simulink model "subsampling2"  (R2021a)
settings: Solver=VariableStepAuto  StartTime=0.0  StopTime=1  MaxStep=1/1e6  RelTol=1e-3
values from neighbouring files (symbols this model uses):
  fnoise = 1e6    (= 1000000)    [subsampling_1.m]    (also in subsampling_2.m; subsampling_3.m = 3000000; unterabtastung_1.m; unterabtastung_2.m)
  fs = 18e3    (= 18000)    [subsampling_1.m]    (also in subsampling_2.m; subsampling_3.m = 450000; unterabtastung_1.m; unterabtastung_2.m)
  fsin = 39e3    (= 39000)    [subsampling_1.m]    (also in subsampling_2.m; subsampling_3.m = 980000; unterabtastung_1.m; unterabtastung_2.m)
undefined symbols (not defined in the file or in its folder): a, b
libraries: simulink x1, dspstat3 x1, dspsigops x1
settings Model: Creator=josef  LastModifiedBy=josef
settings SolverCC: AlgebraicLoopSolver=TrustRegion
settings DataIOCC: ReturnWorkspaceOutputs=off
settings DebuggingCC: SFMachineParentedDataDiag=warning

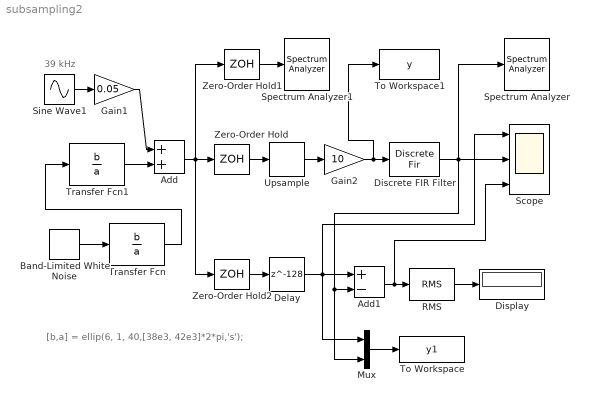
== system subsampling2 ==
  note: [b,a] = ellip(6, 1, 40,[38e3, 42e3]*2*pi,'s');
  note: 39 kHz
  Add : Sum
  Add1 : Sum  Inputs=+-
  Band-Limited White Noise : simulink/Sources/Band-Limited White Noise  Cov=1/fnoise  Ts=1/fnoise  seed=[23341]
  Delay : Delay  DelayLength=128
  Discrete FIR Filter : DiscreteFir  Coefficients=fir1(256,[36, 44]*2e3/(fs*10))
  Display : Display
  Gain1 : Gain  Gain=0.05
  Gain2 : Gain  Gain=10
  Mux : Mux  Inputs=2
  RMS : dspstat3/RMS  run=on  directionMode=Each column  dimension=1  InputProcessing=Columns as channels (frame based)  reset_popup=None
  Scope : Scope  NumInputPorts=3
  Sine Wave1 : Sin  Frequency=2*pi*fsin  SampleTime=0
  Spectrum Analyzer : SpectrumAnalyzer
  Spectrum Analyzer1 : SpectrumAnalyzer
  To Workspace : ToWorkspace  VariableName=y1  SaveFormat=Timeseries  SampleTime=-1
  To Workspace1 : ToWorkspace  VariableName=y  SaveFormat=Timeseries  SampleTime=-1
  Transfer Fcn : TransferFcn  Numerator=b  Denominator=a
  Transfer Fcn1 : TransferFcn  Numerator=b  Denominator=a
  Upsample : dspsigops/Upsample  N=10  phase=0  RateOptions=Allow multirate processing  ic=0  mode=Unused parameter value
  Zero-Order Hold : ZeroOrderHold  SampleTime=1/fs
  Zero-Order Hold1 : ZeroOrderHold  SampleTime=1/(10*fs)
  Zero-Order Hold2 : ZeroOrderHold  SampleTime=1/(10*fs)
  wires:
  Sine Wave1/1 -> Gain1/1
  Add/1 -> Zero-Order Hold2/1, Zero-Order Hold1/1, Zero-Order Hold/1
  Gain1/1 -> Add/1
  Zero-Order Hold/1 -> Upsample/1
  Zero-Order Hold1/1 -> Spectrum Analyzer1/1
  Band-Limited White Noise/1 -> Transfer Fcn/1
  Transfer Fcn/1 -> Transfer Fcn1/1
  Transfer Fcn1/1 -> Add/2
  Upsample/1 -> Gain2/1
  Gain2/1 -> To Workspace1/1, Discrete FIR Filter/1
  Discrete FIR Filter/1 -> Spectrum Analyzer/1, Scope/2, Add1/2, Mux/2
  Zero-Order Hold2/1 -> Delay/1
  Add1/1 -> Scope/3, RMS/1
  RMS/1 -> Display/1
  Delay/1 -> Mux/1, Add1/1, Scope/1
  Mux/1 -> To Workspace/1
